simulink model "QAM"  (R2016a)
settings: Solver=FixedStepDiscrete  StartTime=0.0  StopTime=0.05  FixedStep=1/2000000  RelTol=1e-3
libraries: dsparch4 x7
settings Model: Creator=beac2832  LastModifiedBy=camj3302
settings SolverCC: AutoInsertRateTranBlk=on

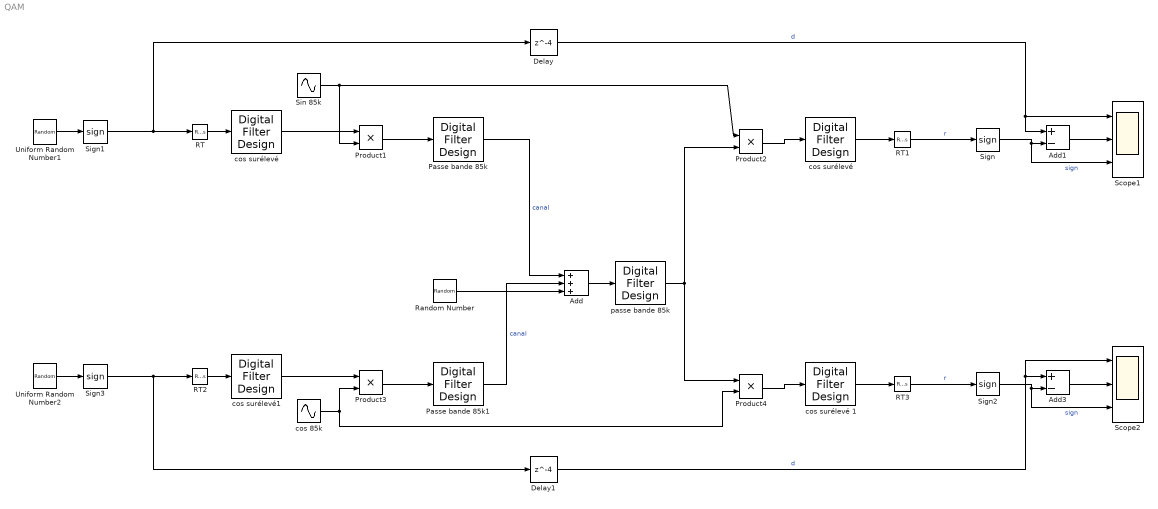
== system QAM ==
  Add : Sum  Inputs=+++
  Add1 : Sum  Inputs=+-
  Add3 : Sum  Inputs=+-
  Delay : Delay  DelayLength=4  InitialCondition=0
  Delay1 : Delay  DelayLength=4  InitialCondition=0
  Passe bande 85k : dsparch4/Digital Filter Design  mwdsp_browser_bugfix_var=off
  Passe bande 85k1 : dsparch4/Digital Filter Design  mwdsp_browser_bugfix_var=off
  Product{1..4} (4 alike) : Product
  RT : RateTransition  OutPortSampleTime=5e-07
  RT1 : RateTransition  OutPortSampleTime=1/1000
  RT2 : RateTransition  OutPortSampleTime=5e-07
  RT3 : RateTransition  OutPortSampleTime=1/1000
  Random Number : RandomNumber  Variance=2  SampleTime=1/2000000
  Scope1 : Scope  NumInputPorts=3
  Scope2 : Scope  NumInputPorts=3
  Sign{,1..3} (4 alike) : Signum
  Sin 85k : Sin  Frequency=85000*2*pi  SampleTime=1/2000000
  Uniform Random Number1 : UniformRandomNumber  SampleTime=1/1000
  Uniform Random Number2 : UniformRandomNumber  SampleTime=1/1000
  cos 85k : Sin  Frequency=85000*2*pi  Phase=pi/2  SampleTime=1/2000000
  cos surélevé : dsparch4/Digital Filter Design  mwdsp_browser_bugfix_var=off
  "cos surélevé " : dsparch4/Digital Filter Design  mwdsp_browser_bugfix_var=off
  cos surélevé 1 : dsparch4/Digital Filter Design  mwdsp_browser_bugfix_var=off
  cos surélevé1 : dsparch4/Digital Filter Design  mwdsp_browser_bugfix_var=off
  passe bande 85k : dsparch4/Digital Filter Design  mwdsp_browser_bugfix_var=off
  wires:
  Product1/1 -> Passe bande 85k/1
  Product2/1 -> "cos surélevé "/1
  Delay/1 -> Scope1/1, Add1/1  "d"
  RT/1 -> cos surélevé/1
  Sign1/1 -> Delay/1, RT/1
  cos surélevé/1 -> Product1/1
  Sin 85k/1 -> Product2/1, Product1/2
  Passe bande 85k/1 -> Add/1  "canal"
  RT1/1 -> Sign/1  "r"
  Add1/1 -> Scope1/2
  Add/1 -> passe bande 85k/1
  "cos surélevé "/1 -> RT1/1
  Sign/1 -> Scope1/3, Add1/2  "sign"
  Uniform Random Number1/1 -> Sign1/1
  Product3/1 -> Passe bande 85k1/1
  Product4/1 -> cos surélevé 1/1
  Delay1/1 -> Scope2/1, Add3/1  "d"
  RT2/1 -> cos surélevé1/1
  Sign3/1 -> Delay1/1, RT2/1
  cos surélevé1/1 -> Product3/1
  cos 85k/1 -> Product3/2, Product4/2
  passe bande 85k/1 -> Product4/1, Product2/2
  Passe bande 85k1/1 -> Add/2  "canal"
  RT3/1 -> Sign2/1  "r"
  Add3/1 -> Scope2/2
  cos surélevé 1/1 -> RT3/1
  Sign2/1 -> Scope2/3, Add3/2  "sign"
  Uniform Random Number2/1 -> Sign3/1
  Random Number/1 -> Add/3
